simulink model "example_1"  (R2020a)
settings: Solver=VariableStepAuto  StartTime=0.0  StopTime=10.0  RelTol=1e-3
settings Model: Creator=Riyansh  LastModifiedBy=Riyansh

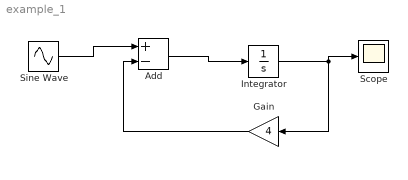
== system example_1 ==
  Add : Sum  Inputs=+-
  Gain : Gain  Gain=4
  Integrator : Integrator
  Scope : Scope
  Sine Wave : Sin  Amplitude=2  Frequency=3  SampleTime=0
  wires:
  Add/1 -> Integrator/1
  Sine Wave/1 -> Add/1
  Integrator/1 -> Scope/1, Gain/1
  Gain/1 -> Add/2
